simulink library "lib_wheel2"  (Simulink 10.1)
settings: Solver=VariableStepAuto  StartTime=0.0  StopTime=10.0  RelTol=1e-3
undefined symbols (not defined in the file or in its folder): lib_help, NOTES, veh_air_density, veh_CD, veh_cg_height, veh_FA, veh_front_wt_frac, veh_gravity, veh_roadwheel_radius, veh_rr_a, veh_rr_alpha, veh_rr_b, veh_rr_beta, veh_rr_c, veh_wheelbase, wh_1st_rrc, wh_2nd_rrc, wh_axle_loss_mass, wh_axle_loss_trq, wh_fa_dl_brake_frac, wh_fa_dl_brake_mph, wh_fa_fric_brake_frac, wh_fa_fric_brake_mph, wh_front_active_bool, wh_inertia, wh_max_front_brake_force, wh_max_rear_brake_force, wh_pressure, wh_radius, wh_rear_active_bool, wh_slip, wh_slip_force_coeff
undefined symbols (not defined in the file): logFlag
libraries: $bdroot x61, lib_vehicle x2, lib_etc x2, lib_controls x2, lib_wheel x1
(part 11 of 13)

== system lib_wheel2/vehicle, wheel, & axle front/rear <wh> 2 axle --> 1 driveline/models and interface/vehicle <veh>/record achieved force outputs ==
  note: local tag
  spd_prev : Inport
  spd : Inport  Port=2
  Gain1 : Gain  Gain=0.5  SaturateOnIntegerOverflow=on
  Product{,1..3} (4 alike) : Product  SaturateOnIntegerOverflow=on
  Sum2 : Sum  SaturateOnIntegerOverflow=on
  enhancedToWorkspace : Subsystem  TreatAsAtomicUnit=on  mask(enhancedToWorkspace){generalName=generalName, specificName=pwr_accel_a, logFlag=logFlag}
      mask prompts: generalName "General Name [char-evaluated]"; specificName "Specific Name [char-literal]"; logFlag "Enable flag (1=on,0=off)"
      mask help: A wrapper for the Simulink "To Workspace" block that allows you to evaluate the name of the variable to log to workspace. This is useful to avoid the double logging errors that occur when you pull in two library models that attempt to log to the same variable.
      mask init:
      | enhancedToWsMaker
      settings: CopyFcn=breakLinkCopyFcn  ParentCloseFcn=breakLinkParCloseFcn
      mask Help:
      | <h2>Enhanced To Workspace Block</h2>
      | <h3>Parameters</h3>
      | <UL>
      | <li><b>General Name:</b> This is the more general name of the variable. Variables are saved to the workspace as <i>generalName_specificName</i>. Note that this is an evaluated variable. If you would like to type in the value directly, it must be surrounded with single quotes. Otherwise you can input the name of a variable containing a char string.</li>
      | <li><b>Specific Name:</b> This is the specific name of the variable. Note that this is input as a char literal (i.e., you don't need quotes).</li>
      | <li><b>Enable Flag:</b> This flag should have the value of 0 or 1. If 0, the variable will not be logged to the workspace. If 1, the variable will be logged. This is done so that variable logging can be turned off to improve speed.</li>
      | </ul>
      | <h3>Overview</h3>
      | <p>The enhanced to workspace block was put together to allow one to dynamically resolve variable names at run time in simulink. This is most powerful when used in conjunction with a masked subsystem to allow multiple instances of that masked subsytem to be used in the same model. The strategy is to set the generalName in the block mask which will allow the block to change the general name for all variable logging on the fly.
      | <h3>Helper Files</h3>
      | <p>Three m-files are required by the enhancedToWorkspace block. These files are located in the &lt; ADVISOR root &gt;/GUI directory :
      | <ul>
      | <li><i>enhancedToWsMaker.m</i> This file runs the mask initialization for the block</li>
      | <li><i>breakLinkCopyFcn.m</i> This file is used by the block callback when the simulink block is copied. It is necessary to break the link to the enhancedToWorkspace similar to the To Workspace block in order for it to be able to configure itself. (Try copying simulink's To Workspace block--it is impossible to make a link)</li>
      | <li><i>breakLinkParCloseFcn.m</i> This file is similar to the breakLinkCopyFcn and is used when a parent system is closed</li>
      | </ul>
      | <hr>
      | 
      | <p>Created 2003-Jan-21, Michael Patrick O'Keefe, NREL</p>
      | 
      | <!--
      | <VARDEF>
      | <H3>var_name</H3>
      | <UL>
      | <LI><B>data type</B> data type here</LI>
      | <LI><B>units</B> units here</LI>
      | <LI><B>vehicle type</B> vehicle type here</LI>
      | <LI><B>description</B> description here</LI>
      | </UL>
      | </VARDEF>
      | -->
      mask Display: disp([generalName,'_',specificName])
  enhancedToWorkspace1 : Subsystem  TreatAsAtomicUnit=on  mask(enhancedToWorkspace){generalName=generalName, specificName=pwr_drag_a, logFlag=logFlag}
      mask prompts: generalName "General Name [char-evaluated]"; specificName "Specific Name [char-literal]"; logFlag "Enable flag (1=on,0=off)"
      mask help: A wrapper for the Simulink "To Workspace" block that allows you to evaluate the name of the variable to log to workspace. This is useful to avoid the double logging errors that occur when you pull in two library models that attempt to log to the same variable.
      mask init:
      | enhancedToWsMaker
      settings: CopyFcn=breakLinkCopyFcn  ParentCloseFcn=breakLinkParCloseFcn
      mask Help:
      | <h2>Enhanced To Workspace Block</h2>
      | <h3>Parameters</h3>
      | <UL>
      | <li><b>General Name:</b> This is the more general name of the variable. Variables are saved to the workspace as <i>generalName_specificName</i>. Note that this is an evaluated variable. If you would like to type in the value directly, it must be surrounded with single quotes. Otherwise you can input the name of a variable containing a char string.</li>
      | <li><b>Specific Name:</b> This is the specific name of the variable. Note that this is input as a char literal (i.e., you don't need quotes).</li>
      | <li><b>Enable Flag:</b> This flag should have the value of 0 or 1. If 0, the variable will not be logged to the workspace. If 1, the variable will be logged. This is done so that variable logging can be turned off to improve speed.</li>
      | </ul>
      | <h3>Overview</h3>
      | <p>The enhanced to workspace block was put together to allow one to dynamically resolve variable names at run time in simulink. This is most powerful when used in conjunction with a masked subsystem to allow multiple instances of that masked subsytem to be used in the same model. The strategy is to set the generalName in the block mask which will allow the block to change the general name for all variable logging on the fly.
      | <h3>Helper Files</h3>
      | <p>Three m-files are required by the enhancedToWorkspace block. These files are located in the &lt; ADVISOR root &gt;/GUI directory :
      | <ul>
      | <li><i>enhancedToWsMaker.m</i> This file runs the mask initialization for the block</li>
      | <li><i>breakLinkCopyFcn.m</i> This file is used by the block callback when the simulink block is copied. It is necessary to break the link to the enhancedToWorkspace similar to the To Workspace block in order for it to be able to configure itself. (Try copying simulink's To Workspace block--it is impossible to make a link)</li>
      | <li><i>breakLinkParCloseFcn.m</i> This file is similar to the breakLinkCopyFcn and is used when a parent system is closed</li>
      | </ul>
      | <hr>
      | 
      | <p>Created 2003-Jan-21, Michael Patrick O'Keefe, NREL</p>
      | 
      | <!--
      | <VARDEF>
      | <H3>var_name</H3>
      | <UL>
      | <LI><B>data type</B> data type here</LI>
      | <LI><B>units</B> units here</LI>
      | <LI><B>vehicle type</B> vehicle type here</LI>
      | <LI><B>description</B> description here</LI>
      | </UL>
      | </VARDEF>
      | -->
      mask Display: disp([generalName,'_',specificName])
  enhancedToWorkspace2 : Subsystem  TreatAsAtomicUnit=on  mask(enhancedToWorkspace){generalName=generalName, specificName=pwr_ascent_a, logFlag=logFlag}
      mask prompts: generalName "General Name [char-evaluated]"; specificName "Specific Name [char-literal]"; logFlag "Enable flag (1=on,0=off)"
      mask help: A wrapper for the Simulink "To Workspace" block that allows you to evaluate the name of the variable to log to workspace. This is useful to avoid the double logging errors that occur when you pull in two library models that attempt to log to the same variable.
      mask init:
      | enhancedToWsMaker
      settings: CopyFcn=breakLinkCopyFcn  ParentCloseFcn=breakLinkParCloseFcn
      mask Help:
      | <h2>Enhanced To Workspace Block</h2>
      | <h3>Parameters</h3>
      | <UL>
      | <li><b>General Name:</b> This is the more general name of the variable. Variables are saved to the workspace as <i>generalName_specificName</i>. Note that this is an evaluated variable. If you would like to type in the value directly, it must be surrounded with single quotes. Otherwise you can input the name of a variable containing a char string.</li>
      | <li><b>Specific Name:</b> This is the specific name of the variable. Note that this is input as a char literal (i.e., you don't need quotes).</li>
      | <li><b>Enable Flag:</b> This flag should have the value of 0 or 1. If 0, the variable will not be logged to the workspace. If 1, the variable will be logged. This is done so that variable logging can be turned off to improve speed.</li>
      | </ul>
      | <h3>Overview</h3>
      | <p>The enhanced to workspace block was put together to allow one to dynamically resolve variable names at run time in simulink. This is most powerful when used in conjunction with a masked subsystem to allow multiple instances of that masked subsytem to be used in the same model. The strategy is to set the generalName in the block mask which will allow the block to change the general name for all variable logging on the fly.
      | <h3>Helper Files</h3>
      | <p>Three m-files are required by the enhancedToWorkspace block. These files are located in the &lt; ADVISOR root &gt;/GUI directory :
      | <ul>
      | <li><i>enhancedToWsMaker.m</i> This file runs the mask initialization for the block</li>
      | <li><i>breakLinkCopyFcn.m</i> This file is used by the block callback when the simulink block is copied. It is necessary to break the link to the enhancedToWorkspace similar to the To Workspace block in order for it to be able to configure itself. (Try copying simulink's To Workspace block--it is impossible to make a link)</li>
      | <li><i>breakLinkParCloseFcn.m</i> This file is similar to the breakLinkCopyFcn and is used when a parent system is closed</li>
      | </ul>
      | <hr>
      | 
      | <p>Created 2003-Jan-21, Michael Patrick O'Keefe, NREL</p>
      | 
      | <!--
      | <VARDEF>
      | <H3>var_name</H3>
      | <UL>
      | <LI><B>data type</B> data type here</LI>
      | <LI><B>units</B> units here</LI>
      | <LI><B>vehicle type</B> vehicle type here</LI>
      | <LI><B>description</B> description here</LI>
      | </UL>
      | </VARDEF>
      | -->
      mask Display: disp([generalName,'_',specificName])
  enhancedToWorkspace3 : Subsystem  TreatAsAtomicUnit=on  mask(enhancedToWorkspace){generalName=generalName, specificName=pwr_rr_a, logFlag=logFlag}
      mask prompts: generalName "General Name [char-evaluated]"; specificName "Specific Name [char-literal]"; logFlag "Enable flag (1=on,0=off)"
      mask help: A wrapper for the Simulink "To Workspace" block that allows you to evaluate the name of the variable to log to workspace. This is useful to avoid the double logging errors that occur when you pull in two library models that attempt to log to the same variable.
      mask init:
      | enhancedToWsMaker
      settings: CopyFcn=breakLinkCopyFcn  ParentCloseFcn=breakLinkParCloseFcn
      mask Help:
      | <h2>Enhanced To Workspace Block</h2>
      | <h3>Parameters</h3>
      | <UL>
      | <li><b>General Name:</b> This is the more general name of the variable. Variables are saved to the workspace as <i>generalName_specificName</i>. Note that this is an evaluated variable. If you would like to type in the value directly, it must be surrounded with single quotes. Otherwise you can input the name of a variable containing a char string.</li>
      | <li><b>Specific Name:</b> This is the specific name of the variable. Note that this is input as a char literal (i.e., you don't need quotes).</li>
      | <li><b>Enable Flag:</b> This flag should have the value of 0 or 1. If 0, the variable will not be logged to the workspace. If 1, the variable will be logged. This is done so that variable logging can be turned off to improve speed.</li>
      | </ul>
      | <h3>Overview</h3>
      | <p>The enhanced to workspace block was put together to allow one to dynamically resolve variable names at run time in simulink. This is most powerful when used in conjunction with a masked subsystem to allow multiple instances of that masked subsytem to be used in the same model. The strategy is to set the generalName in the block mask which will allow the block to change the general name for all variable logging on the fly.
      | <h3>Helper Files</h3>
      | <p>Three m-files are required by the enhancedToWorkspace block. These files are located in the &lt; ADVISOR root &gt;/GUI directory :
      | <ul>
      | <li><i>enhancedToWsMaker.m</i> This file runs the mask initialization for the block</li>
      | <li><i>breakLinkCopyFcn.m</i> This file is used by the block callback when the simulink block is copied. It is necessary to break the link to the enhancedToWorkspace similar to the To Workspace block in order for it to be able to configure itself. (Try copying simulink's To Workspace block--it is impossible to make a link)</li>
      | <li><i>breakLinkParCloseFcn.m</i> This file is similar to the breakLinkCopyFcn and is used when a parent system is closed</li>
      | </ul>
      | <hr>
      | 
      | <p>Created 2003-Jan-21, Michael Patrick O'Keefe, NREL</p>
      | 
      | <!--
      | <VARDEF>
      | <H3>var_name</H3>
      | <UL>
      | <LI><B>data type</B> data type here</LI>
      | <LI><B>units</B> units here</LI>
      | <LI><B>vehicle type</B> vehicle type here</LI>
      | <LI><B>description</B> description here</LI>
      | </UL>
      | </VARDEF>
      | -->
      mask Display: disp([generalName,'_',specificName])
  force req'd to accelerate (N) : $bdroot/vehicle, wheel, & axle front//rear <wh>/models and interface/vehicle <veh>/force req'd to accelerate (N)
      settings: RTWFcnNameOpts=Auto  RTWFileNameOpts=Auto
  force req'd to ascend (N) : $bdroot/vehicle, wheel, & axle front//rear <wh>/models and interface/vehicle <veh>/force req'd to ascend (N)
      settings: RTWFcnNameOpts=Auto  RTWFileNameOpts=Auto
  force req'd to overcome aerodynamic drag (N) : $bdroot/vehicle, wheel, & axle front//rear <wh>/models and interface/vehicle <veh>/force req'd to overcome aerodynamic drag (N)
      settings: RTWFcnNameOpts=Auto  RTWFileNameOpts=Auto
  rolling resistance force : Subsystem  BlockChoice=force req'd to overcome rolling resistance (N)
      settings: AttributesFormatString=%<BlockChoice>  TemplateBlock=lib_wheel2/Submodels/rolling resistance force  MemberBlocks=force req'd to overcome rolling resistance (N),force req'd to overcome rolling resistance (N) j2452
  tag scope: veh_pwr_accel_a=scoped, veh_pwr_ascent_a=scoped, veh_pwr_drag_a=scoped, veh_pwr_rr_a=scoped
  wires:
  Sum2/1 -> Gain1/1
  spd/1 -> Sum2/1, force req'd to accelerate (N)/1
  spd_prev/1 -> Sum2/2, force req'd to accelerate (N)/2
  force req'd to overcome aerodynamic drag (N)/1 -> Product1/1
  force req'd to ascend (N)/1 -> Product2/1
  rolling resistance force/1(Fr (N)) -> Product3/1
  force req'd to accelerate (N)/1 -> Product/1
  Product/1 -> [veh_pwr_accel_a], enhancedToWorkspace/1(In1)
  Product1/1 -> [veh_pwr_drag_a], enhancedToWorkspace1/1(In1)
  [vel_ave] -> Product/2
  [vel_ave] -> Product1/2
  [vel_ave] -> Product2/2
  Product2/1 -> [veh_pwr_ascent_a], enhancedToWorkspace2/1(In1)
  [vel_ave] -> Product3/2
  Product3/1 -> [veh_pwr_rr_a], enhancedToWorkspace3/1(In1)
  Gain1/1 -> force req'd to ascend (N)/1, rolling resistance force/1(average vehicle speed over time step (m/s)), [vel_ave], force req'd to overcome aerodynamic drag (N)/1

== system lib_wheel2/vehicle, wheel, & axle front/rear <wh> 2 axle --> 1 driveline/models and interface/vehicle <veh>/rolling resistance force ==
  average vehicle speed over time step (m/s) : Inport
  force req'd to overcome rolling resistance (N) : $bdroot/Submodels/force req'd to overcome rolling resistance (N)
      settings: RTWFcnNameOpts=Auto  RTWFileNameOpts=Auto
  Fr (N) : Outport
  wires:
  force req'd to overcome rolling resistance (N)/1 -> Fr (N)/1
  average vehicle speed over time step (m/s)/1 -> force req'd to overcome rolling resistance (N)/1

== system lib_wheel2/vehicle, wheel, & axle front/rear <wh> 2 axle --> 1 driveline/models and interface/vehicle <veh>/vehicle speed ==
  vehicle speed at beginning of time step (m/s) : Inport
  "available tractive force and linear speed (N), (m/s)" : Inport  Port=2
  vehicle speed (m/s) : $bdroot/Submodels/vehicle speed (m//s)
      settings: RTWFcnNameOpts=Auto  RTWFileNameOpts=Auto
  vehicle speed achievable at end of time step (m/s) : Outport
  wires:
  vehicle speed (m/s)/1 -> vehicle speed achievable at end of time step (m/s)/1
  "available tractive force and linear speed (N), (m/s)"/1 -> vehicle speed (m/s)/2
  vehicle speed at beginning of time step (m/s)/1 -> vehicle speed (m/s)/1

== system lib_wheel2/vehicle, wheel, & axle front/rear <wh> 2 axle --> 1 driveline/models and interface/wheel and axle  front/rear <wh>/Block NOTES ==
  note: This block determines the required axle torque and speed given the tractive force and
      | speed required to meet the trace in the top blocks, and determines the available tractive
      | force and possible vehicle speed given the drivetrain-input torque and rotational speed
      | in the bottom blocks.  The "wheel control" blocks apply the braking strategy and ensure
      | that accelerations beyond the capability of the tires are not requested.

== system lib_wheel2/vehicle, wheel, & axle front/rear <wh> 2 axle --> 1 driveline/models and interface/wheel and axle  front/rear <wh>/effect of  inertia (Nm) ==
  note: This block computes the torque required to overcome the inertia of the
      | wheels and axle.
  axle input speed (rad/s) : Inport
  Constant : Constant  Value=wh_inertia
  Product : Product  SaturateOnIntegerOverflow=on
  d/dt : Derivative
  inertia torque (Nm) : Outport  InitialOutput=0
  wires:
  d/dt/1 -> Product/1
  axle input speed (rad/s)/1 -> d/dt/1
  Constant/1 -> Product/2
  Product/1 -> inertia torque (Nm)/1

== system lib_wheel2/vehicle, wheel, & axle front/rear <wh> 2 axle --> 1 driveline/models and interface/wheel and axle  front/rear <wh>/enhancedToWorkspace ==
  In1 : Inport
  To Workspace : ToWorkspace  VariableName=wh_rear_spd_a  SampleTime=-1
  wires:
  In1/1 -> To Workspace/1

== system lib_wheel2/vehicle, wheel, & axle front/rear <wh> 2 axle --> 1 driveline/models and interface/wheel and axle  front/rear <wh>/enhancedToWorkspace1 ==
  In1 : Inport
  To Workspace : ToWorkspace  VariableName=wh_wt_front_axle  SampleTime=-1
  wires:
  In1/1 -> To Workspace/1

== system lib_wheel2/vehicle, wheel, & axle front/rear <wh> 2 axle --> 1 driveline/models and interface/wheel and axle  front/rear <wh>/enhancedToWorkspace10 ==
  In1 : Inport
  To Workspace : ToWorkspace  VariableName=wh_trq_r  SampleTime=-1
  wires:
  In1/1 -> To Workspace/1

== system lib_wheel2/vehicle, wheel, & axle front/rear <wh> 2 axle --> 1 driveline/models and interface/wheel and axle  front/rear <wh>/enhancedToWorkspace11 ==
  In1 : Inport
  To Workspace : ToWorkspace  VariableName=wh_rear_brake_a  SampleTime=-1
  wires:
  In1/1 -> To Workspace/1

== system lib_wheel2/vehicle, wheel, & axle front/rear <wh> 2 axle --> 1 driveline/models and interface/wheel and axle  front/rear <wh>/enhancedToWorkspace12 ==
  In1 : Inport
  To Workspace : ToWorkspace  VariableName=wh_front_brake_a  SampleTime=-1
  wires:
  In1/1 -> To Workspace/1

== system lib_wheel2/vehicle, wheel, & axle front/rear <wh> 2 axle --> 1 driveline/models and interface/wheel and axle  front/rear <wh>/enhancedToWorkspace2 ==
  In1 : Inport
  To Workspace : ToWorkspace  VariableName=wh_front_traction_ratio  SampleTime=-1
  wires:
  In1/1 -> To Workspace/1

== system lib_wheel2/vehicle, wheel, & axle front/rear <wh> 2 axle --> 1 driveline/models and interface/wheel and axle  front/rear <wh>/enhancedToWorkspace3 ==
  In1 : Inport
  To Workspace : ToWorkspace  VariableName=wh_wt_rear_axle  SampleTime=-1
  wires:
  In1/1 -> To Workspace/1

== system lib_wheel2/vehicle, wheel, & axle front/rear <wh> 2 axle --> 1 driveline/models and interface/wheel and axle  front/rear <wh>/enhancedToWorkspace4 ==
  In1 : Inport
  To Workspace : ToWorkspace  VariableName=wh_trq_a  SampleTime=-1
  wires:
  In1/1 -> To Workspace/1

== system lib_wheel2/vehicle, wheel, & axle front/rear <wh> 2 axle --> 1 driveline/models and interface/wheel and axle  front/rear <wh>/enhancedToWorkspace5 ==
  In1 : Inport
  To Workspace : ToWorkspace  VariableName=wh_spd_a  SampleTime=-1
  wires:
  In1/1 -> To Workspace/1

== system lib_wheel2/vehicle, wheel, & axle front/rear <wh> 2 axle --> 1 driveline/models and interface/wheel and axle  front/rear <wh>/enhancedToWorkspace6 ==
  In1 : Inport
  To Workspace : ToWorkspace  VariableName=wh_rear_trq_a  SampleTime=-1
  wires:
  In1/1 -> To Workspace/1

== system lib_wheel2/vehicle, wheel, & axle front/rear <wh> 2 axle --> 1 driveline/models and interface/wheel and axle  front/rear <wh>/enhancedToWorkspace7 ==
  In1 : Inport
  To Workspace : ToWorkspace  VariableName=wh_rear_spd_r  SampleTime=-1
  wires:
  In1/1 -> To Workspace/1

== system lib_wheel2/vehicle, wheel, & axle front/rear <wh> 2 axle --> 1 driveline/models and interface/wheel and axle  front/rear <wh>/enhancedToWorkspace8 ==
  In1 : Inport
  To Workspace : ToWorkspace  VariableName=wh_rear_trq_r  SampleTime=-1
  wires:
  In1/1 -> To Workspace/1

== system lib_wheel2/vehicle, wheel, & axle front/rear <wh> 2 axle --> 1 driveline/models and interface/wheel and axle  front/rear <wh>/enhancedToWorkspace9 ==
  In1 : Inport
  To Workspace : ToWorkspace  VariableName=wh_spd_r  SampleTime=-1
  wires:
  In1/1 -> To Workspace/1

== system lib_wheel2/vehicle, wheel, & axle front/rear <wh> 2 axle --> 1 driveline/models and interface/wheel and axle  front/rear <wh>/front brake ==
  F_brake : Inport
  Constant : Constant  Value=wh_max_front_brake_force
  Terminator : Terminator
  F_brake_max : Outport  InitialOutput=0
  wires:
  F_brake/1 -> Terminator/1
  Constant/1 -> F_brake_max/1

== system lib_wheel2/vehicle, wheel, & axle front/rear <wh> 2 axle --> 1 driveline/models and interface/wheel and axle  front/rear <wh>/front force ==
  In1 : Inport
  In2 : Inport  Port=2
  Product1 : Product  SaturateOnIntegerOverflow=on
  Sum2 : Sum  Inputs=-+  SaturateOnIntegerOverflow=on
  brake request  controller interface : Subsystem
  enhancedToWorkspace11 : Subsystem  TreatAsAtomicUnit=on  mask(enhancedToWorkspace){generalName=generalName01, specificName=front_brake_r, logFlag=logFlag}
      mask prompts: generalName "General Name [char-evaluated]"; specificName "Specific Name [char-literal]"; logFlag "Enable flag (1=on,0=off)"
      mask help: A wrapper for the Simulink "To Workspace" block that allows you to evaluate the name of the variable to log to workspace. This is useful to avoid the double logging errors that occur when you pull in two library models that attempt to log to the same variable.
      mask init:
      | enhancedToWsMaker
      settings: CopyFcn=breakLinkCopyFcn  ParentCloseFcn=breakLinkParCloseFcn
      mask Help:
      | <h2>Enhanced To Workspace Block</h2>
      | <h3>Parameters</h3>
      | <UL>
      | <li><b>General Name:</b> This is the more general name of the variable. Variables are saved to the workspace as <i>generalName_specificName</i>. Note that this is an evaluated variable. If you would like to type in the value directly, it must be surrounded with single quotes. Otherwise you can input the name of a variable containing a char string.</li>
      | <li><b>Specific Name:</b> This is the specific name of the variable. Note that this is input as a char literal (i.e., you don't need quotes).</li>
      | <li><b>Enable Flag:</b> This flag should have the value of 0 or 1. If 0, the variable will not be logged to the workspace. If 1, the variable will be logged. This is done so that variable logging can be turned off to improve speed.</li>
      | </ul>
      | <h3>Overview</h3>
      | <p>The enhanced to workspace block was put together to allow one to dynamically resolve variable names at run time in simulink. This is most powerful when used in conjunction with a masked subsystem to allow multiple instances of that masked subsytem to be used in the same model. The strategy is to set the generalName in the block mask which will allow the block to change the general name for all variable logging on the fly.
      | <h3>Helper Files</h3>
      | <p>Three m-files are required by the enhancedToWorkspace block. These files are located in the &lt; ADVISOR root &gt;/GUI directory :
      | <ul>
      | <li><i>enhancedToWsMaker.m</i> This file runs the mask initialization for the block</li>
      | <li><i>breakLinkCopyFcn.m</i> This file is used by the block callback when the simulink block is copied. It is necessary to break the link to the enhancedToWorkspace similar to the To Workspace block in order for it to be able to configure itself. (Try copying simulink's To Workspace block--it is impossible to make a link)</li>
      | <li><i>breakLinkParCloseFcn.m</i> This file is similar to the breakLinkCopyFcn and is used when a parent system is closed</li>
      | </ul>
      | <hr>
      | 
      | <p>Created 2003-Jan-21, Michael Patrick O'Keefe, NREL</p>
      | 
      | <!--
      | <VARDEF>
      | <H3>var_name</H3>
      | <UL>
      | <LI><B>data type</B> data type here</LI>
      | <LI><B>units</B> units here</LI>
      | <LI><B>vehicle type</B> vehicle type here</LI>
      | <LI><B>description</B> description here</LI>
      | </UL>
      | </VARDEF>
      | -->
      mask Display: disp([generalName,'_',specificName])
  tractive torque req/d of drivetrain (Nm) : Gain  Gain=wh_radius  SaturateOnIntegerOverflow=on
  Out1 : Outport
  wires:
  brake request  controller interface/1(F_front_brake_req) -> Sum2/1, enhancedToWorkspace11/1(In1)
  Sum2/1 -> tractive torque req/d of drivetrain (Nm)/1
  Product1/1 -> Sum2/2
  In1/1 -> Product1/1
  In2/1 -> Product1/2
  tractive torque req/d of drivetrain (Nm)/1 -> Out1/1

== system lib_wheel2/vehicle, wheel, & axle front/rear <wh> 2 axle --> 1 driveline/models and interface/wheel and axle  front/rear <wh>/front/rear brake controller interface (achievable) ==
  F_drivetrain_ach : Inport
  w_wheel_ach : Inport  Port=2
  F_rear_drivetrain_ach : Inport  Port=3
  F_max_front_brake : Inport  Port=4
  F_max_rear_brake : Inport  Port=5
  F_front_brake : Outport  InitialOutput=0
  F_rear_brake : Outport  Port=2  InitialOutput=0
  tag scope: F_drivetrain_ach=scoped, F_max_front_brake=scoped, F_max_rear_brake=scoped, F_rear_drivetrain_ach=scoped, w_wheel_ach=scoped
  wires:
  [F_rear_brake] -> F_rear_brake/1
  [F_front_brake] -> F_front_brake/1
  w_wheel_ach/1 -> [w_wheel_ach]
  F_drivetrain_ach/1 -> [F_drivetrain_ach]
  F_max_front_brake/1 -> [F_max_front_brake]
  F_max_rear_brake/1 -> [F_max_rear_brake]
  F_rear_drivetrain_ach/1 -> [F_rear_drivetrain_ach]

== system lib_wheel2/vehicle, wheel, & axle front/rear <wh> 2 axle --> 1 driveline/models and interface/wheel and axle  front/rear <wh>/help ==

== system lib_wheel2/vehicle, wheel, & axle front/rear <wh> 2 axle --> 1 driveline/models and interface/wheel and axle  front/rear <wh>/limits and losses diagnostics ==
  speed : Inport
  front brake : Inport  Port=2
  front brake max : Inport  Port=3
  rear brake max : Inport  Port=4
  rear brake : Inport  Port=5
  Gain : Gain  Gain=-1  SaturateOnIntegerOverflow=on
  Logical Operator : Logic  Operator=OR
  Product : Product  SaturateOnIntegerOverflow=on
  Relational Operator1 : RelationalOperator  Operator===  RndMeth=Nearest  InputSameDT=on
  Relational Operator2 : RelationalOperator  Operator===  RndMeth=Nearest  InputSameDT=on
  Sum3 : Sum  SaturateOnIntegerOverflow=on
  enhancedToWorkspace : Subsystem  TreatAsAtomicUnit=on  mask(enhancedToWorkspace){generalName=generalName01, specificName=brake_loss_pwr, logFlag=logFlag}
      mask prompts: generalName "General Name [char-evaluated]"; specificName "Specific Name [char-literal]"; logFlag "Enable flag (1=on,0=off)"
      mask help: A wrapper for the Simulink "To Workspace" block that allows you to evaluate the name of the variable to log to workspace. This is useful to avoid the double logging errors that occur when you pull in two library models that attempt to log to the same variable.
      mask init:
      | enhancedToWsMaker
      settings: CopyFcn=breakLinkCopyFcn  ParentCloseFcn=breakLinkParCloseFcn
      mask Help:
      | <h2>Enhanced To Workspace Block</h2>
      | <h3>Parameters</h3>
      | <UL>
      | <li><b>General Name:</b> This is the more general name of the variable. Variables are saved to the workspace as <i>generalName_specificName</i>. Note that this is an evaluated variable. If you would like to type in the value directly, it must be surrounded with single quotes. Otherwise you can input the name of a variable containing a char string.</li>
      | <li><b>Specific Name:</b> This is the specific name of the variable. Note that this is input as a char literal (i.e., you don't need quotes).</li>
      | <li><b>Enable Flag:</b> This flag should have the value of 0 or 1. If 0, the variable will not be logged to the workspace. If 1, the variable will be logged. This is done so that variable logging can be turned off to improve speed.</li>
      | </ul>
      | <h3>Overview</h3>
      | <p>The enhanced to workspace block was put together to allow one to dynamically resolve variable names at run time in simulink. This is most powerful when used in conjunction with a masked subsystem to allow multiple instances of that masked subsytem to be used in the same model. The strategy is to set the generalName in the block mask which will allow the block to change the general name for all variable logging on the fly.
      | <h3>Helper Files</h3>
      | <p>Three m-files are required by the enhancedToWorkspace block. These files are located in the &lt; ADVISOR root &gt;/GUI directory :
      | <ul>
      | <li><i>enhancedToWsMaker.m</i> This file runs the mask initialization for the block</li>
      | <li><i>breakLinkCopyFcn.m</i> This file is used by the block callback when the simulink block is copied. It is necessary to break the link to the enhancedToWorkspace similar to the To Workspace block in order for it to be able to configure itself. (Try copying simulink's To Workspace block--it is impossible to make a link)</li>
      | <li><i>breakLinkParCloseFcn.m</i> This file is similar to the breakLinkCopyFcn and is used when a parent system is closed</li>
      | </ul>
      | <hr>
      | 
      | <p>Created 2003-Jan-21, Michael Patrick O'Keefe, NREL</p>
      | 
      | <!--
      | <VARDEF>
      | <H3>var_name</H3>
      | <UL>
      | <LI><B>data type</B> data type here</LI>
      | <LI><B>units</B> units here</LI>
      | <LI><B>vehicle type</B> vehicle type here</LI>
      | <LI><B>description</B> description here</LI>
      | </UL>
      | </VARDEF>
      | -->
      mask Display: disp([generalName,'_',specificName])
  tag scope: brake_limited=scoped
  wires:
  Gain/1 -> Product/2
  Sum3/1 -> Gain/1
  Product/1 -> enhancedToWorkspace/1(In1)
  Logical Operator/1 -> [brake_limited]
  Relational Operator1/1 -> Logical Operator/1
  Relational Operator2/1 -> Logical Operator/2
  speed/1 -> Product/1
  front brake/1 -> Sum3/1, Relational Operator1/1
  front brake max/1 -> Relational Operator1/2
  rear brake max/1 -> Relational Operator2/1
  rear brake/1 -> Sum3/2, Relational Operator2/2

== system lib_wheel2/vehicle, wheel, & axle front/rear <wh> 2 axle --> 1 driveline/models and interface/wheel and axle  front/rear <wh>/loss (Nm) ==
  note: The loss torque is zero when the axle is not turning.
  axle speed (rad/s) : Inport
  Constant : Constant  Value=0
  Switch : Switch  Threshold=eps  SaturateOnIntegerOverflow=on  InputSameDT=on
  current veh mass : $bdroot/Submodels/current veh mass
      settings: RTWFcnNameOpts=Auto  RTWFileNameOpts=Auto
  wheel & axle bearing drag (Nm) : Lookup  InputValues=wh_axle_loss_mass  Table=wh_axle_loss_trq  SaturateOnIntegerOverflow=on
  drag torque (Nm) : Outport  InitialOutput=0
  wires:
  current veh mass/1 -> wheel & axle bearing drag (Nm)/1
  Switch/1 -> drag torque (Nm)/1
  axle speed (rad/s)/1 -> Switch/2
  Constant/1 -> Switch/3
  wheel & axle bearing drag (Nm)/1 -> Switch/1

== system lib_wheel2/vehicle, wheel, & axle front/rear <wh> 2 axle --> 1 driveline/models and interface/wheel and axle  front/rear <wh>/rear brake ==
  F_brake : Inport
  Constant : Constant  Value=wh_max_rear_brake_force
  Terminator : Terminator
  F_brake_max : Outport  InitialOutput=0
  wires:
  Constant/1 -> F_brake_max/1
  F_brake/1 -> Terminator/1

== system lib_wheel2/vehicle, wheel, & axle front/rear <wh> 2 axle --> 1 driveline/models and interface/wheel and axle  front/rear <wh>/rear force ==
  In1 : Inport
  In2 : Inport  Port=2
  Product2 : Product  SaturateOnIntegerOverflow=on
  Sum1 : Sum  Inputs=-+  SaturateOnIntegerOverflow=on
  Sum4 : Sum  Inputs=-+  SaturateOnIntegerOverflow=on
  brake request controller interface1 : Subsystem
  enhancedToWorkspace : Subsystem  TreatAsAtomicUnit=on  mask(enhancedToWorkspace){generalName=generalName01, specificName=rear_brake_r, logFlag=logFlag}
      mask prompts: generalName "General Name [char-evaluated]"; specificName "Specific Name [char-literal]"; logFlag "Enable flag (1=on,0=off)"
      mask help: A wrapper for the Simulink "To Workspace" block that allows you to evaluate the name of the variable to log to workspace. This is useful to avoid the double logging errors that occur when you pull in two library models that attempt to log to the same variable.
      mask init:
      | enhancedToWsMaker
      settings: CopyFcn=breakLinkCopyFcn  ParentCloseFcn=breakLinkParCloseFcn
      mask Help:
      | <h2>Enhanced To Workspace Block</h2>
      | <h3>Parameters</h3>
      | <UL>
      | <li><b>General Name:</b> This is the more general name of the variable. Variables are saved to the workspace as <i>generalName_specificName</i>. Note that this is an evaluated variable. If you would like to type in the value directly, it must be surrounded with single quotes. Otherwise you can input the name of a variable containing a char string.</li>
      | <li><b>Specific Name:</b> This is the specific name of the variable. Note that this is input as a char literal (i.e., you don't need quotes).</li>
      | <li><b>Enable Flag:</b> This flag should have the value of 0 or 1. If 0, the variable will not be logged to the workspace. If 1, the variable will be logged. This is done so that variable logging can be turned off to improve speed.</li>
      | </ul>
      | <h3>Overview</h3>
      | <p>The enhanced to workspace block was put together to allow one to dynamically resolve variable names at run time in simulink. This is most powerful when used in conjunction with a masked subsystem to allow multiple instances of that masked subsytem to be used in the same model. The strategy is to set the generalName in the block mask which will allow the block to change the general name for all variable logging on the fly.
      | <h3>Helper Files</h3>
      | <p>Three m-files are required by the enhancedToWorkspace block. These files are located in the &lt; ADVISOR root &gt;/GUI directory :
      | <ul>
      | <li><i>enhancedToWsMaker.m</i> This file runs the mask initialization for the block</li>
      | <li><i>breakLinkCopyFcn.m</i> This file is used by the block callback when the simulink block is copied. It is necessary to break the link to the enhancedToWorkspace similar to the To Workspace block in order for it to be able to configure itself. (Try copying simulink's To Workspace block--it is impossible to make a link)</li>
      | <li><i>breakLinkParCloseFcn.m</i> This file is similar to the breakLinkCopyFcn and is used when a parent system is closed</li>
      | </ul>
      | <hr>
      | 
      | <p>Created 2003-Jan-21, Michael Patrick O'Keefe, NREL</p>
      | 
      | <!--
      | <VARDEF>
      | <H3>var_name</H3>
      | <UL>
      | <LI><B>data type</B> data type here</LI>
      | <LI><B>units</B> units here</LI>
      | <LI><B>vehicle type</B> vehicle type here</LI>
      | <LI><B>description</B> description here</LI>
      | </UL>
      | </VARDEF>
      | -->
      mask Display: disp([generalName,'_',specificName])
  tractive torque req/d of drivetrain (Nm)1 : Gain  Gain=wh_radius  SaturateOnIntegerOverflow=on
  Out1 : Outport
  wires:
  brake request controller interface1/1(F_rear_brake_req) -> Sum4/1, enhancedToWorkspace/1(In1)
  Sum4/1 -> tractive torque req/d of drivetrain (Nm)1/1
  tractive torque req/d of drivetrain (Nm)1/1 -> Out1/1
  In1/1 -> Product2/1, Sum1/2
  In2/1 -> Product2/2
  Product2/1 -> Sum1/1
  Sum1/1 -> Sum4/2

== system lib_wheel2/vehicle, wheel, & axle front/rear <wh> 2 axle --> 1 driveline/models and interface/wheel and axle  front/rear <wh>/tire slip model (m/s) ==
  note: See note regarding sum in backward path
  weight borne  by front axle (N) : Inport
  total tractive  force available (N) : Inport  Port=2
  axle speed available (rad/s) : Inport  Port=3
  axle speed req'd (rad/s) : Inport  Port=4
  vehicle speed required (m/s) : Inport  Port=5
  weight borne by  rear axle (N) : Inport  Port=6
  front fraction : Inport  Port=7
  Abs1 : Abs  SaturateOnIntegerOverflow=on
  Block NOTES : Subsystem
      mask Display: disp('Block\nNOTES')
  Constant : Constant  Value=1e-3
  Constant5 : Constant
  Constant6 : Constant  Value=wh_radius
  Fcn : Fcn  Expr=1/u
  Relational Operator1 : RelationalOperator  Operator=>  RndMeth=Nearest  InputSameDT=on
  Sum1 : Sum  Inputs=+-  SaturateOnIntegerOverflow=on
  Sum2 : Sum  SaturateOnIntegerOverflow=on
  Sum3 : Sum  SaturateOnIntegerOverflow=on
  Sum4 : Sum  Inputs=-+  SaturateOnIntegerOverflow=on
  Switch1 : Switch  Threshold=eps  SaturateOnIntegerOverflow=on  InputSameDT=on
  front axle : Subsystem
  front frac : Product  SaturateOnIntegerOverflow=on
  rear axle : Subsystem
  vehicle speed (m/s) : Product  Inputs=3  SaturateOnIntegerOverflow=on
  possible vehicle speed (m/s) : Outport  InitialOutput=0
  tag scope: veh_spd_a_rec=scoped
  wires:
  Sum3/1 -> Fcn/1
  Fcn/1 -> vehicle speed (m/s)/1
  Constant5/1 -> Sum3/2
  axle speed available (rad/s)/1 -> Sum4/1, vehicle speed (m/s)/2
  Constant6/1 -> vehicle speed (m/s)/3
  Relational Operator1/1 -> Switch1/2
  vehicle speed required (m/s)/1 -> Switch1/3
  Sum4/1 -> Abs1/1
  axle speed req'd (rad/s)/1 -> Sum4/2
  Constant/1 -> Relational Operator1/2
  Abs1/1 -> Relational Operator1/1
  weight borne  by front axle (N)/1 -> front axle/1(In1)
  Switch1/1 -> possible vehicle speed (m/s)/1
  vehicle speed (m/s)/1 -> Switch1/1, [veh_spd_a_rec]
  weight borne by  rear axle (N)/1 -> rear axle/1(In1)
  total tractive  force available (N)/1 -> front frac/1, Sum1/1
  front fraction/1 -> front frac/2
  front frac/1 -> front axle/2(In2), Sum1/2
  Sum1/1 -> rear axle/2(In2)
  front axle/1(Out1) -> Sum2/1
  rear axle/1(Out1) -> Sum2/2
  Sum2/1 -> Sum3/1

== system lib_wheel2/vehicle, wheel, & axle front/rear <wh> 2 axle --> 1 driveline/models and interface/wheel and axle  front/rear <wh>/tire slip model (rad/s) ==
  note: Slip is defined as s=(omega*r - v) / v.  The one-to-one mapping of slip to normalized
      | tractive force, F_tract/W_front_axle, up to the maximum, is stored in the variables
      | "wh_slip" and "wh_slip_force_coeff."
  note: This block implements the effects of finite tire slip
      | (with respect to the road) on the vehicle speed/wheel speed relationship.
  note: Question: for front and rear, is it the sum of or min/max? tm:020703
  total tractive  force requested (N) : Inport
  requested time-step average vehicle speed (m/s) : Inport  Port=2
  weight borne by front axle (N) : Inport  Port=3
  weight borne by  rear axle (N)1 : Inport  Port=4
  front traction ratio : Inport  Port=5
  Constant5 : Constant
  Constant6 : Constant  Value=1/wh_radius
  Sum1 : Sum  Inputs=+-  SaturateOnIntegerOverflow=on
  Sum2 : Sum  SaturateOnIntegerOverflow=on
  Sum3 : Sum  SaturateOnIntegerOverflow=on
  enhancedToWorkspace : Subsystem  TreatAsAtomicUnit=on  mask(enhancedToWorkspace){generalName=generalName01, specificName=slip_r, logFlag=logFlag}
      mask prompts: generalName "General Name [char-evaluated]"; specificName "Specific Name [char-literal]"; logFlag "Enable flag (1=on,0=off)"
      mask help: A wrapper for the Simulink "To Workspace" block that allows you to evaluate the name of the variable to log to workspace. This is useful to avoid the double logging errors that occur when you pull in two library models that attempt to log to the same variable.
      mask init:
      | enhancedToWsMaker
      settings: CopyFcn=breakLinkCopyFcn  ParentCloseFcn=breakLinkParCloseFcn
      mask Help:
      | <h2>Enhanced To Workspace Block</h2>
      | <h3>Parameters</h3>
      | <UL>
      | <li><b>General Name:</b> This is the more general name of the variable. Variables are saved to the workspace as <i>generalName_specificName</i>. Note that this is an evaluated variable. If you would like to type in the value directly, it must be surrounded with single quotes. Otherwise you can input the name of a variable containing a char string.</li>
      | <li><b>Specific Name:</b> This is the specific name of the variable. Note that this is input as a char literal (i.e., you don't need quotes).</li>
      | <li><b>Enable Flag:</b> This flag should have the value of 0 or 1. If 0, the variable will not be logged to the workspace. If 1, the variable will be logged. This is done so that variable logging can be turned off to improve speed.</li>
      | </ul>
      | <h3>Overview</h3>
      | <p>The enhanced to workspace block was put together to allow one to dynamically resolve variable names at run time in simulink. This is most powerful when used in conjunction with a masked subsystem to allow multiple instances of that masked subsytem to be used in the same model. The strategy is to set the generalName in the block mask which will allow the block to change the general name for all variable logging on the fly.
      | <h3>Helper Files</h3>
      | <p>Three m-files are required by the enhancedToWorkspace block. These files are located in the &lt; ADVISOR root &gt;/GUI directory :
      | <ul>
      | <li><i>enhancedToWsMaker.m</i> This file runs the mask initialization for the block</li>
      | <li><i>breakLinkCopyFcn.m</i> This file is used by the block callback when the simulink block is copied. It is necessary to break the link to the enhancedToWorkspace similar to the To Workspace block in order for it to be able to configure itself. (Try copying simulink's To Workspace block--it is impossible to make a link)</li>
      | <li><i>breakLinkParCloseFcn.m</i> This file is similar to the breakLinkCopyFcn and is used when a parent system is closed</li>
      | </ul>
      | <hr>
      | 
      | <p>Created 2003-Jan-21, Michael Patrick O'Keefe, NREL</p>
      | 
      | <!--
      | <VARDEF>
      | <H3>var_name</H3>
      | <UL>
      | <LI><B>data type</B> data type here</LI>
      | <LI><B>units</B> units here</LI>
      | <LI><B>vehicle type</B> vehicle type here</LI>
      | <LI><B>description</B> description here</LI>
      | </UL>
      | </VARDEF>
      | -->
      mask Display: disp([generalName,'_',specificName])
  front frac : Product  SaturateOnIntegerOverflow=on
  front slip : Subsystem
  rear slip : Subsystem
  wheel speed (rad/s) : Product  Inputs=3  SaturateOnIntegerOverflow=on
  slip-augmented rotational speed (rad/s) : Outport  InitialOutput=0
  wires:
  weight borne by front axle (N)/1 -> front slip/1(In1)
  requested time-step average vehicle speed (m/s)/1 -> wheel speed (rad/s)/1
  Constant6/1 -> wheel speed (rad/s)/3
  Sum3/1 -> wheel speed (rad/s)/2
  Constant5/1 -> Sum3/2
  wheel speed (rad/s)/1 -> slip-augmented rotational speed (rad/s)/1
  front frac/1 -> Sum1/2, front slip/2(In2)
  total tractive  force requested (N)/1 -> front frac/1, Sum1/1
  front traction ratio/1 -> front frac/2
  Sum1/1 -> rear slip/2(In2)
  weight borne by  rear axle (N)1/1 -> rear slip/1(In1)
  front slip/1(Out1) -> Sum2/1
  rear slip/1(Out1) -> Sum2/2
  Sum2/1 -> Sum3/1, enhancedToWorkspace/1(In1)

== system lib_wheel2/vehicle, wheel, & axle front/rear <wh> 2 axle --> 1 driveline/models and interface/wheel and axle  front/rear <wh>/traction controller interface ==
  F_req : Inport
  v_ave_req : Inport  Port=2
  F_req_limited : Outport  InitialOutput=0
  v_req_limited : Outport  Port=2  InitialOutput=0
  wt_front_axle : Outport  Port=3  InitialOutput=0
  wt_rear_axle : Outport  Port=4  InitialOutput=0
  front_traction_ratio : Outport  Port=5  InitialOutput=0
  tag scope: F_req=scoped, v_ave_req=scoped
  wires:
  [F_req_limited] -> F_req_limited/1
  [v_req_limited] -> v_req_limited/1
  [wt_front_axle] -> wt_front_axle/1
  F_req/1 -> [F_req]
  v_ave_req/1 -> [v_ave_req]
  [wt_rear_axle] -> wt_rear_axle/1
  [front_traction_ratio] -> front_traction_ratio/1

== system lib_wheel2/development/wheel and axle  front/rear <wh>/wheel & axle model & interface/wheel model/Block NOTES ==
  note: This block determines the required axle torque and speed given the tractive force and
      | speed required to meet the trace in the top blocks, and determines the available tractive
      | force and possible vehicle speed given the drivetrain-input torque and rotational speed
      | in the bottom blocks.  The "wheel control" blocks apply the braking strategy and ensure
      | that accelerations beyond the capability of the tires are not requested.

== system lib_wheel2/development/wheel and axle  front/rear <wh>/wheel & axle model & interface/wheel model/effect of  inertia (Nm) ==
  note: This block computes the torque required to overcome the inertia of the
      | wheels and axle.
  axle input speed (rad/s) : Inport
  Constant : Constant  Value=wh_inertia
  Product : Product  SaturateOnIntegerOverflow=on
  d/dt : Derivative
  inertia torque (Nm) : Outport  InitialOutput=0
  wires:
  d/dt/1 -> Product/1
  axle input speed (rad/s)/1 -> d/dt/1
  Constant/1 -> Product/2
  Product/1 -> inertia torque (Nm)/1

== system lib_wheel2/development/wheel and axle  front/rear <wh>/wheel & axle model & interface/wheel model/enhancedToWorkspace ==
  In1 : Inport
  To Workspace : ToWorkspace  VariableName=wh_rear_spd_a  SampleTime=-1
  wires:
  In1/1 -> To Workspace/1

== system lib_wheel2/development/wheel and axle  front/rear <wh>/wheel & axle model & interface/wheel model/enhancedToWorkspace1 ==
  In1 : Inport
  To Workspace : ToWorkspace  VariableName=wh_rear_trq_a  SampleTime=-1
  wires:
  In1/1 -> To Workspace/1

== system lib_wheel2/development/wheel and axle  front/rear <wh>/wheel & axle model & interface/wheel model/enhancedToWorkspace10 ==
  In1 : Inport
  To Workspace : ToWorkspace  VariableName=wh_trq_r  SampleTime=-1
  wires:
  In1/1 -> To Workspace/1

== system lib_wheel2/development/wheel and axle  front/rear <wh>/wheel & axle model & interface/wheel model/enhancedToWorkspace11 ==
  In1 : Inport
  To Workspace : ToWorkspace  VariableName=wh_rear_spd_r  SampleTime=-1
  wires:
  In1/1 -> To Workspace/1

== system lib_wheel2/development/wheel and axle  front/rear <wh>/wheel & axle model & interface/wheel model/enhancedToWorkspace12 ==
  In1 : Inport
  To Workspace : ToWorkspace  VariableName=wh_rear_trq_r  SampleTime=-1
  wires:
  In1/1 -> To Workspace/1

== system lib_wheel2/development/wheel and axle  front/rear <wh>/wheel & axle model & interface/wheel model/enhancedToWorkspace2 ==
  In1 : Inport
  To Workspace : ToWorkspace  VariableName=wh_rear_brake_a  SampleTime=-1
  wires:
  In1/1 -> To Workspace/1

== system lib_wheel2/development/wheel and axle  front/rear <wh>/wheel & axle model & interface/wheel model/enhancedToWorkspace3 ==
  In1 : Inport
  To Workspace : ToWorkspace  VariableName=wh_front_brake_a  SampleTime=-1
  wires:
  In1/1 -> To Workspace/1

== system lib_wheel2/development/wheel and axle  front/rear <wh>/wheel & axle model & interface/wheel model/enhancedToWorkspace4 ==
  In1 : Inport
  To Workspace : ToWorkspace  VariableName=wh_spd_a  SampleTime=-1
  wires:
  In1/1 -> To Workspace/1

== system lib_wheel2/development/wheel and axle  front/rear <wh>/wheel & axle model & interface/wheel model/enhancedToWorkspace5 ==
  In1 : Inport
  To Workspace : ToWorkspace  VariableName=wh_trq_a  SampleTime=-1
  wires:
  In1/1 -> To Workspace/1

== system lib_wheel2/development/wheel and axle  front/rear <wh>/wheel & axle model & interface/wheel model/enhancedToWorkspace6 ==
  In1 : Inport
  To Workspace : ToWorkspace  VariableName=wh_front_traction_ratio  SampleTime=-1
  wires:
  In1/1 -> To Workspace/1

== system lib_wheel2/development/wheel and axle  front/rear <wh>/wheel & axle model & interface/wheel model/enhancedToWorkspace7 ==
  In1 : Inport
  To Workspace : ToWorkspace  VariableName=wh_wt_rear_axle  SampleTime=-1
  wires:
  In1/1 -> To Workspace/1

== system lib_wheel2/development/wheel and axle  front/rear <wh>/wheel & axle model & interface/wheel model/enhancedToWorkspace8 ==
  In1 : Inport
  To Workspace : ToWorkspace  VariableName=wh_wt_front_axle  SampleTime=-1
  wires:
  In1/1 -> To Workspace/1
